simulink model "stand_IM_LSP_1"  (R2024a)
settings: Solver=ode45  StartTime=0.0  StopTime=10.0  RelTol=1e-3  EnableMultiTasking=on
values from neighbouring files (symbols this model uses):
  pp = 2    [stand_final.m]
libraries: General x36, MotorControl x5, Math x4, Basic x2, Filter x2, StateControl x1, Control x1
settings Model: Creator=hgrabner  LastModifiedBy=adminLab
settings SolverCC: AlgebraicLoopSolver=TrustRegion
settings DataIOCC: LimitDataPoints=on  SaveFormat=Array  SignalLoggingSaveFormat=ModelDataLogs  ReturnWorkspaceOutputs=off
settings OptimizationCC: ExpressionDepthLimit=2147483647  InitFltsAndDblsToZero=on  LifeSpan=inf
settings DebuggingCC: UnderspecifiedInitializationDetection=Classic  MergeDetectMultiDrivingBlocksExec=none  SolverPrmCheckMsg=warning  FcnCallInpInsideContextMsg=warning  UnconnectedInputMsg=warning  UnconnectedOutputMsg=warning  UnconnectedLineMsg=warning  StateNameClashWarn=warning  SFUnexpectedBacktrackingDiag=warning  SFNoUnconditionalDefaultTransitionDiag=warning  SFExecutionAtInitializationDiag=none  ArithmeticOperatorsInVariantConditions=warning
settings HardwareCC: ProdBitPerPointer=32  ProdBitPerSizeT=32  ProdBitPerPtrDiffT=32  ProdLargestAtomicFloat=None  ProdIntDivRoundTo=Undefined  ProdEndianess=Unspecified  ProdWordSize=32  ProdHWDeviceType=32-bit Generic
settings ModelReferenceCC: EnableRefExpFcnMdlSchedulingChecks=on  PropagateSignalLabelsOutOfModel=off
settings SFSimCC: SimUseLocalCustomCode=off  CustomCodeUndefinedFunction=UseInterfaceOnly
settings RTWCC: RTWUseLocalCustomCode=off  GPUComputeCapability=3.5  DLArmComputeVersion=19.05
settings CodeAppCC: StateflowObjectComments=on
settings GRTTargetCC: TargetLangStandard=C89/C90 (ANSI)  CombineOutputUpdateFcns=off  GRTInterface=on
settings ConfigComp: CovMetricSettings=dw  CovSaveCumulativeToWorkspaceVar=on  CovSaveSingleToWorkspaceVar=on  CovExternalEMLEnable=off

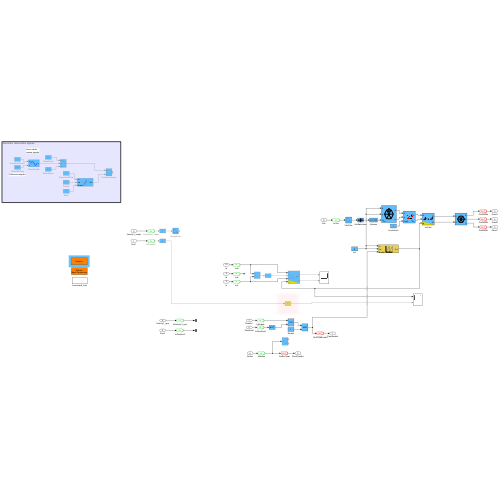
[thumbnail: Simulink's stored preview of the top-level diagram]
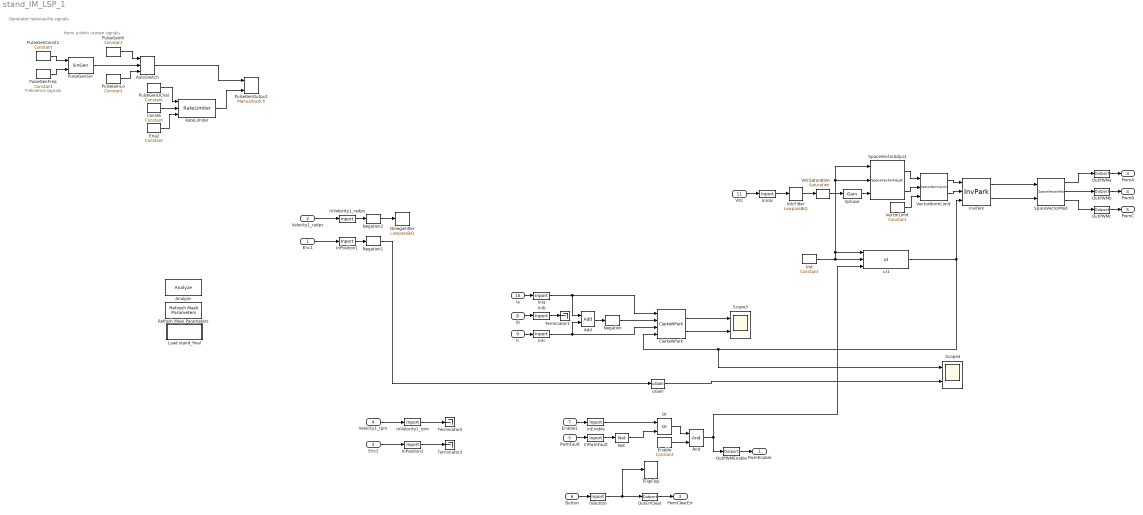
== system stand_IM_LSP_1 ==
  note: Frekvence signalu
  note: Generator testovaciho signalu
  note: Horni a dolni
      | uroven signalu
  Enc1 : Inport
  Velocity1_radps : Inport  Port=2
  Enc2 : Inport  Port=3
  Velocity1_rpm : Inport  Port=4
  PwmFault : Inport  Port=5
  Button : Inport  Port=6
  Enable1 : Inport  Port=7
  Ib : Inport  Port=8
  Ic : Inport  Port=9
  Ia : Inport  Port=10
  Vdc : Inport  Port=11
  Add : Math/Add  M2CAutoParam_UsedImplementation=32 Bit Floating Point  x2c_cfg_enableStaticId=off  x2c_cfg_staticId=1  x2c_cfg_enableCot=off  BlockName=Add
      settings: SourceProductName=X2C Math
  Analyze : Basic/Analyze
      settings: SourceProductName=X2C Basic
  And : General/And  M2CAutoParam_UsedImplementation=Boolean  x2c_cfg_enableStaticId=off  x2c_cfg_staticId=1  x2c_cfg_enableCot=off  BlockName=And
      settings: SourceProductName=X2C General
  AutoSwitch : General/AutoSwitch  Thresh_up=0.01  Thresh_down=-0.01  M2CAutoParam_UsedImplementation=32 Bit Floating Point  x2c_cfg_enableStaticId=off  x2c_cfg_staticId=1  x2c_cfg_enableCot=off  BlockName=AutoSwitch
      settings: SourceProductName=X2C General
  ClarkeNPark : MotorControl/ClarkeNPark  M2CAutoParam_UsedImplementation=32 Bit Floating Point  x2c_cfg_enableStaticId=off  x2c_cfg_staticId=1  x2c_cfg_enableCot=off  BlockName=ClarkeNPark
      settings: SourceProductName=X2C MotorControl
  Const6 : General/Constant  Value=0  M2CAutoParam_UsedImplementation=32 Bit Floating Point  x2c_cfg_enableStaticId=off  x2c_cfg_staticId=1  x2c_cfg_enableCot=off  BlockName=Constant
      settings: SourceProductName=X2C General
  Ena2 : General/Constant  Value=1  M2CAutoParam_UsedImplementation=Boolean  x2c_cfg_enableStaticId=off  x2c_cfg_staticId=1  x2c_cfg_enableCot=off  BlockName=Constant
      settings: SourceProductName=X2C General
  Enable : General/Constant  Value=1  M2CAutoParam_UsedImplementation=Boolean  x2c_cfg_enableStaticId=off  x2c_cfg_staticId=1  x2c_cfg_enableCot=off  BlockName=Constant
      settings: SourceProductName=X2C General
  InButton : General/Inport  DataType=bool  ts_fact=1.0  x2c_cfg_enableStaticId=off  x2c_cfg_staticId=0  BlockName=Inport  gain=1  offset=0
      settings: SourceProductName=X2C General
  InEnable : General/Inport  DataType=bool  ts_fact=1.0  x2c_cfg_enableStaticId=off  x2c_cfg_staticId=0  BlockName=Inport  gain=1  offset=0
      settings: SourceProductName=X2C General
  InIa : General/Inport  DataType=float32  ts_fact=1.0  x2c_cfg_enableStaticId=off  x2c_cfg_staticId=0  BlockName=Inport  gain=1  offset=0
      settings: SourceProductName=X2C General
  InIb : General/Inport  DataType=float32  ts_fact=1.0  x2c_cfg_enableStaticId=off  x2c_cfg_staticId=0  BlockName=Inport  gain=1  offset=0
      settings: SourceProductName=X2C General
  InIc : General/Inport  DataType=float32  ts_fact=1.0  x2c_cfg_enableStaticId=off  x2c_cfg_staticId=0  BlockName=Inport  gain=1  offset=0
      settings: SourceProductName=X2C General
  InPosition1 : General/Inport  DataType=float32  ts_fact=20  x2c_cfg_enableStaticId=off  x2c_cfg_staticId=0  BlockName=Inport  gain=1  offset=0
      settings: SourceProductName=X2C General
  InPosition2 : General/Inport  DataType=float32  ts_fact=1.0  x2c_cfg_enableStaticId=off  x2c_cfg_staticId=0  BlockName=Inport  gain=1  offset=0
      settings: SourceProductName=X2C General
  InPwmFault : General/Inport  DataType=bool  ts_fact=1.0  x2c_cfg_enableStaticId=off  x2c_cfg_staticId=0  BlockName=Inport  gain=1  offset=0
      settings: SourceProductName=X2C General
  InVdc : General/Inport  DataType=float32  ts_fact=1.0  x2c_cfg_enableStaticId=off  x2c_cfg_staticId=0  BlockName=Inport  gain=1  offset=0
      settings: SourceProductName=X2C General
  InVelocity1_radps : General/Inport  DataType=float32  ts_fact=20  x2c_cfg_enableStaticId=off  x2c_cfg_staticId=0  BlockName=Inport  gain=1  offset=0
      settings: SourceProductName=X2C General
  InVelocity1_rpm : General/Inport  DataType=float32  ts_fact=1.0  x2c_cfg_enableStaticId=off  x2c_cfg_staticId=0  BlockName=Inport  gain=1  offset=0
      settings: SourceProductName=X2C General
  Init : General/Constant  Value=0  M2CAutoParam_UsedImplementation=32 Bit Floating Point  x2c_cfg_enableStaticId=off  x2c_cfg_staticId=1  x2c_cfg_enableCot=off  BlockName=Constant
      settings: SourceProductName=X2C General
  InvPark : MotorControl/InvPark  M2CAutoParam_UsedImplementation=32 Bit Floating Point  x2c_cfg_enableStaticId=off  x2c_cfg_staticId=1  x2c_cfg_enableCot=off  BlockName=InvPark
      settings: SourceProductName=X2C MotorControl
  Load stand_final : Subsystem  InitFcn=stand_final
      settings: OpenFcn=stand_final
      mask DialogControl Control2 Prompt: Load stand_final
  Negation : Math/Negation  M2CAutoParam_UsedImplementation=32 Bit Floating Point  x2c_cfg_enableStaticId=off  x2c_cfg_staticId=1  x2c_cfg_enableCot=off  BlockName=Negation
      settings: SourceProductName=X2C Math
  Negation1 : Math/Negation  M2CAutoParam_UsedImplementation=32 Bit Floating Point  x2c_cfg_enableStaticId=off  x2c_cfg_staticId=1  x2c_cfg_enableCot=off  BlockName=Negation
      settings: SourceProductName=X2C Math
  Negation2 : Math/Negation  M2CAutoParam_UsedImplementation=32 Bit Floating Point  x2c_cfg_enableStaticId=off  x2c_cfg_staticId=1  x2c_cfg_enableCot=off  BlockName=Negation
      settings: SourceProductName=X2C Math
  Not : General/Not  M2CAutoParam_UsedImplementation=Boolean  x2c_cfg_enableStaticId=off  x2c_cfg_staticId=1  x2c_cfg_enableCot=off  BlockName=Not
      settings: SourceProductName=X2C General
  OmegaFilter : Filter/LowpassBiQ  characteristic=Chebyshev II  fc=200  rp=1  rs=20  ts_fact=20  M2CAutoParam_UsedImplementation=32 Bit Floating Point  x2c_cfg_enableStaticId=off  x2c_cfg_staticId=1  x2c_cfg_enableCot=off  BlockName=LowpassBiQ
      settings: SourceProductName=X2C Filter
  Or : General/Or  M2CAutoParam_UsedImplementation=Boolean  x2c_cfg_enableStaticId=off  x2c_cfg_staticId=1  x2c_cfg_enableCot=off  BlockName=Or
      settings: SourceProductName=X2C General
  OutErrClear : General/Outport  DataType=bool  ts_fact=1.0  x2c_cfg_enableStaticId=off  x2c_cfg_staticId=0  BlockName=Outport  gain=1  offset=0
      settings: SourceProductName=X2C General
  OutPWMEnable : General/Outport  DataType=bool  ts_fact=1.0  x2c_cfg_enableStaticId=off  x2c_cfg_staticId=0  BlockName=Outport  gain=1  offset=0
      settings: SourceProductName=X2C General
  OutPWMa : General/Outport  DataType=float32  ts_fact=1.0  x2c_cfg_enableStaticId=off  x2c_cfg_staticId=0  BlockName=Outport  gain=1  offset=0
      settings: SourceProductName=X2C General
  OutPWMb : General/Outport  DataType=float32  ts_fact=1.0  x2c_cfg_enableStaticId=off  x2c_cfg_staticId=0  BlockName=Outport  gain=1  offset=0
      settings: SourceProductName=X2C General
  OutPWMc : General/Outport  DataType=float32  ts_fact=1.0  x2c_cfg_enableStaticId=off  x2c_cfg_staticId=0  BlockName=Outport  gain=1  offset=0
      settings: SourceProductName=X2C General
  PulseGenConst1 : General/Constant  Value=1  M2CAutoParam_UsedImplementation=32 Bit Floating Point  x2c_cfg_enableStaticId=off  x2c_cfg_staticId=1  x2c_cfg_enableCot=off  BlockName=Constant
      settings: SourceProductName=X2C General
  PulseGenDCVal : General/Constant  Value=0  M2CAutoParam_UsedImplementation=32 Bit Floating Point  x2c_cfg_enableStaticId=off  x2c_cfg_staticId=1  x2c_cfg_enableCot=off  BlockName=Constant
      settings: SourceProductName=X2C General
  PulseGenFreq : General/Constant  Value=0.25  M2CAutoParam_UsedImplementation=32 Bit Floating Point  x2c_cfg_enableStaticId=off  x2c_cfg_staticId=1  x2c_cfg_enableCot=off  BlockName=Constant
      settings: SourceProductName=X2C General
  PulseGenHi : General/Constant  Value=30  M2CAutoParam_UsedImplementation=32 Bit Floating Point  x2c_cfg_enableStaticId=off  x2c_cfg_staticId=1  x2c_cfg_enableCot=off  BlockName=Constant
      settings: SourceProductName=X2C General
  PulseGenLo : General/Constant  Value=20  M2CAutoParam_UsedImplementation=32 Bit Floating Point  x2c_cfg_enableStaticId=off  x2c_cfg_staticId=1  x2c_cfg_enableCot=off  BlockName=Constant
      settings: SourceProductName=X2C General
  PulseGenOutput : General/ManualSwitch  Toggle=1  M2CAutoParam_UsedImplementation=32 Bit Floating Point  x2c_cfg_enableStaticId=off  x2c_cfg_staticId=1  x2c_cfg_enableCot=off  BlockName=ManualSwitch
      settings: SourceProductName=X2C General
  PulseGenSin : General/SinGen  fmax=1000.0  Phase=0.0  ts_fact=20  M2CAutoParam_UsedImplementation=32 Bit Floating Point  x2c_cfg_enableStaticId=off  x2c_cfg_staticId=1  x2c_cfg_enableCot=off  BlockName=SinGen  Offset=0.0
      settings: SourceProductName=X2C General
  RateLimiter : General/RateLimiter  Tr=0.1  Tf=0.1  ts_fact=20  M2CAutoParam_UsedImplementation=32 Bit Floating Point  x2c_cfg_enableStaticId=off  x2c_cfg_staticId=1  x2c_cfg_enableCot=off  BlockName=RateLimiter
      settings: SourceProductName=X2C General
  Refresh Mask Parameters : Basic/Refresh Mask Parameters
      settings: SourceProductName=X2C Basic
  Scope3 : Scope  NumInputPorts=2
  Scope4 : Scope  NumInputPorts=2
  SpaceVectorAdjust : MotorControl/SpaceVectorAdjust  M2CAutoParam_UsedImplementation=32 Bit Floating Point  x2c_cfg_enableStaticId=off  x2c_cfg_staticId=1  x2c_cfg_enableCot=off  BlockName=SpaceVectorAdjust
      settings: SourceProductName=X2C MotorControl
  SpaceVectorMod : MotorControl/SpaceVectorMod  method=Alternating reversing  M2CAutoParam_UsedImplementation=32 Bit Floating Point  x2c_cfg_enableStaticId=off  x2c_cfg_staticId=1  x2c_cfg_enableCot=off  BlockName=SpaceVectorMod
      settings: SourceProductName=X2C MotorControl
  TFlipFlop : StateControl/TFlipFlop  M2CAutoParam_UsedImplementation=Boolean  x2c_cfg_enableStaticId=off  x2c_cfg_staticId=1  x2c_cfg_enableCot=off  BlockName=TFlipFlop
      settings: SourceProductName=X2C StateControl
  Terminator2 : Terminator
  Terminator3 : Terminator
  Terminator5 : Terminator
  VdcFilter : Filter/LowpassBiQ  characteristic=Chebyshev II  fc=10  rp=1  rs=20  ts_fact=1  M2CAutoParam_UsedImplementation=32 Bit Floating Point  x2c_cfg_enableStaticId=off  x2c_cfg_staticId=1  x2c_cfg_enableCot=off  BlockName=LowpassBiQ
      settings: SourceProductName=X2C Filter
  VdcSaturation : General/Saturation  max=60  min=10  M2CAutoParam_UsedImplementation=32 Bit Floating Point  x2c_cfg_enableStaticId=off  x2c_cfg_staticId=1  x2c_cfg_enableCot=off  BlockName=Saturation
      settings: SourceProductName=X2C General
  VectorLimit : General/Constant  Value=1  M2CAutoParam_UsedImplementation=32 Bit Floating Point  x2c_cfg_enableStaticId=off  x2c_cfg_staticId=1  x2c_cfg_enableCot=off  BlockName=Constant
      settings: SourceProductName=X2C General
  VectorNormLimit : MotorControl/VectorNormLimit  M2CAutoParam_UsedImplementation=32 Bit Floating Point  x2c_cfg_enableStaticId=off  x2c_cfg_staticId=1  x2c_cfg_enableCot=off  BlockName=VectorNormLimit
      settings: SourceProductName=X2C MotorControl
  Vphase : General/Gain  Gain=1/sqrt(3)  M2CAutoParam_UsedImplementation=32 Bit Floating Point  x2c_cfg_enableStaticId=off  x2c_cfg_staticId=1  x2c_cfg_enableCot=off  BlockName=Gain
      settings: SourceProductName=X2C General
  uGain : General/uGain  Gain=pp  M2CAutoParam_UsedImplementation=32 Bit Floating Point  x2c_cfg_enableStaticId=off  x2c_cfg_staticId=1  x2c_cfg_enableCot=off  BlockName=uGain
      settings: SourceProductName=X2C General
  uI1 : Control/uI  Ki=1  ts_fact=1.0  M2CAutoParam_UsedImplementation=32 Bit Floating Point  x2c_cfg_enableStaticId=off  x2c_cfg_staticId=1  x2c_cfg_enableCot=off  BlockName=uI
      settings: SourceProductName=X2C Control
  PwmEnable : Outport
  PwmClearErr : Outport  Port=2
  PwmA : Outport  Port=3
  PwmB : Outport  Port=4
  PwmC : Outport  Port=5
  wires:
  InIb/1 -> Terminator3/1
  uI1/1 -> InvPark/3, Scope4/1, ClarkeNPark/4
  InvPark/1 -> SpaceVectorMod/1
  uGain/1 -> Scope4/2
  InvPark/2 -> SpaceVectorMod/2
  VectorNormLimit/1 -> InvPark/1
  Init/1 -> uI1/2, uI1/1, SpaceVectorAdjust/2, SpaceVectorAdjust/1
  ClarkeNPark/1 -> Scope3/1
  ClarkeNPark/2 -> Scope3/2
  VectorNormLimit/2 -> InvPark/2
  InVdc/1 -> VdcFilter/1
  Add/1 -> Negation/1
  Negation/1 -> ClarkeNPark/2
  SpaceVectorMod/2 -> OutPWMb/1
  InIa/1 -> ClarkeNPark/1, Add/1
  SpaceVectorMod/1 -> OutPWMa/1
  SpaceVectorMod/3 -> OutPWMc/1
  InIc/1 -> ClarkeNPark/3, Add/2
  Negation1/1 -> uGain/1
  InButton/1 -> TFlipFlop/1, OutErrClear/1
  InPwmFault/1 -> Not/1
  Not/1 -> Or/2
  InEnable/1 -> Or/1
  Or/1 -> And/1
  And/1 -> uI1/3, OutPWMEnable/1
  Enable/1 -> And/2
  Velocity1_radps/1 -> InVelocity1_radps/1
  InPosition1/1 -> Negation1/1
  Enc1/1 -> InPosition1/1
  InVelocity1_rpm/1 -> Terminator5/1
  Enc2/1 -> InPosition2/1
  Velocity1_rpm/1 -> InVelocity1_rpm/1
  InPosition2/1 -> Terminator2/1
  PwmFault/1 -> InPwmFault/1
  Enable1/1 -> InEnable/1
  Button/1 -> InButton/1
  Ic/1 -> InIc/1
  Ib/1 -> InIb/1
  Ia/1 -> InIa/1
  Vdc/1 -> InVdc/1
  OutErrClear/1 -> PwmClearErr/1
  OutPWMEnable/1 -> PwmEnable/1
  OutPWMb/1 -> PwmB/1
  OutPWMc/1 -> PwmC/1
  OutPWMa/1 -> PwmA/1
  InVelocity1_radps/1 -> Negation2/1
  Negation2/1 -> OmegaFilter/1
  VdcFilter/1 -> VdcSaturation/1
  VdcSaturation/1 -> Vphase/1
  SpaceVectorAdjust/2 -> VectorNormLimit/2
  SpaceVectorAdjust/1 -> VectorNormLimit/1
  Vphase/1 -> SpaceVectorAdjust/3
  VectorLimit/1 -> VectorNormLimit/3
  RateLimiter/1 -> PulseGenOutput/2
  PulseGenFreq/1 -> PulseGenSin/2
  PulseGenLo/1 -> AutoSwitch/3
  PulseGenHi/1 -> AutoSwitch/1
  AutoSwitch/1 -> PulseGenOutput/1
  Const6/1 -> RateLimiter/2
  PulseGenConst1/1 -> PulseGenSin/1
  PulseGenSin/1 -> AutoSwitch/2
  Ena2/1 -> RateLimiter/3
  PulseGenDCVal/1 -> RateLimiter/1

== system stand_IM_LSP_1/Load stand_final ==
